simulink model "sampleModel7293_pp_1_1"  (R2018a)
settings: Solver=VariableStepAuto  StartTime=0.0  StopTime=10.0  RelTol=1e-3
undefined symbols (not defined in the file): DiscIntNeverNeededParam
libraries: simulink x367
(part 5 of 12)

== system sampleModel7293_pp_1_1/cfblk209 ==
  cfblk1 : Inport
  Action Port : ActionPort  ActionType=else
  cfblk10 : Subsystem  TreatAsAtomicUnit=on
  cfblk11 : Delay
  cfblk12 : Subsystem  TreatAsAtomicUnit=on
  cfblk13 : Delay
  cfblk3 : DiscreteTransferFcn
  cfblk4 : Subsystem  TreatAsAtomicUnit=on
  cfblk5 : simulink/Continuous/PID Controller (2DOF)  Controller=PID  TimeDomain=Discrete-time  SampleTime=-1  IntegratorMethod=Forward Euler  FilterMethod=Forward Euler  Form=Parallel  UseFilter=on  ControllerParametersSource=internal  P=1  I=1  D=0  N=100  b=1  c=1  InitialConditionSource=internal  InitialConditionForIntegrator=0  InitialConditionForFilter=0  ExternalReset=none  LimitOutput=off  UpperSaturationLimit=inf  LowerSaturationLimit=-inf  LinearizeAsGain=off  AntiWindupMode=none  Kb=1  TrackingMode=off  Kt=1  PParamMin=[]  PParamMax=[]  IParamMin=[]  IParamMax=[]  DParamMin=[]  DParamMax=[]  NParamMin=[]  NParamMax=[]  bParamMin=[]  bParamMax=[]  cParamMin=[]  cParamMax=[]  KbParamMin=[]  KbParamMax=[]  KtParamMin=[]  KtParamMax=[]  POutMin=[]  POutMax=[]  IOutMin=[]  IOutMax=[]  DOutMin=[]  DOutMax=[]  NOutMin=[]  NOutMax=[]  bOutMin=[]  bOutMax=[]  cOutMin=[]  cOutMax=[]  KbOutMin=[]  KbOutMax=[]  KtOutMin=[]  KtOutMax=[]  IntegratorOutMin=[]  IntegratorOutMax=[]  FilterOutMin=[]  FilterOutMax=[]  SumOutMin=[]  SumOutMax=[]  Sum1OutMin=[]  Sum1OutMax=[]  Sum2OutMin=[]  Sum2OutMax=[]  Sum3OutMin=[]  Sum3OutMax=[]  SumI1OutMin=[]  SumI1OutMax=[]  SumI2OutMin=[]  SumI2OutMax=[]  SumI3OutMin=[]  SumI3OutMax=[]  SumDOutMin=[]  SumDOutMax=[]  SaturationOutMin=[]  SaturationOutMax=[]  IntegratorContinuousStateAttributes=''  IntegratorStateMustResolveToSignalObject=off  IntegratorRTWStateStorageClass=Auto  FilterContinuousStateAttributes=''  FilterStateMustResolveToSignalObject=off  FilterRTWStateStorageClass=Auto  DifferentiatorICPrevScaledInput=0  DifferentiatorOutMin=[]  DifferentiatorOutMax=[]  FilterDiffOutCoefMin=[]  FilterDiffOutCoefMax=[]  SumDenOutMin=[]  SumDenOutMax=[]  SumNumOutMin=[]  SumNumOutMax=[]  ReciprocalOutMin=[]  ReciprocalOutMax=[]  DivideOutMin=[]  DivideOutMax=[]  TunerSelectOption=Transfer Function Based (PID Tuner App)
  cfblk6 : Subsystem  TreatAsAtomicUnit=on
  cfblk7 : simulink/Discrete/Difference  ICPrevInput=0.0  OutMin=[]  OutMax=[]  OutDataTypeStr=double  OutputDataTypeScalingMode=double  OutDataType=fixdt(1, 16)  OutScaling=2^-10  DoSatur=off
  cfblk8 : If  SampleTime=1
  cfblk9 : Subsystem  TreatAsAtomicUnit=on
  cyemi_{1328..1329,1341..1352} (14 alike) : DataTypeConversion  OutDataTypeStr=double
  emi_1702 : Subsystem  TreatAsAtomicUnit=on
  emi_1704 : If  IfExpression=0 <= u1
  emi_1705 : DataTypeConversion  OutDataTypeStr=double
  emi_1908 : Subsystem  TreatAsAtomicUnit=on
  emi_1910 : If  IfExpression=0 <= u1
  emi_1911 : DataTypeConversion  OutDataTypeStr=double
  emi_783 : Subsystem  TreatAsAtomicUnit=on
  emi_785 : If  IfExpression=0 <= u1
  emi_786 : DataTypeConversion  OutDataTypeStr=double
  cfblk2 : Outport
  wires:
  cfblk10/1(cfblk2) -> cfblk2/1
  cfblk7/1 -> cyemi_1342/1, cyemi_1343/1
  cfblk8/1 -> cfblk9/Action
  cfblk8/2 -> cfblk10/Action
  cyemi_1328/1 -> cfblk10/1(cfblk1)
  cyemi_1329/1 -> cfblk10/2(cfblk12)
  cfblk13/1 -> cyemi_1329/1, emi_786/1
  cyemi_1341/1 -> cfblk11/1
  cfblk5/1 -> cyemi_1341/1
  cyemi_1343/1 -> cfblk13/1
  cyemi_1344/1 -> cfblk3/1
  cfblk9/1(cfblk2) -> cyemi_1344/1
  cyemi_1346/1 -> cfblk5/1
  cfblk3/1 -> cyemi_1346/1
  cyemi_1347/1 -> cfblk5/2
  cfblk9/2(cfblk16) -> cyemi_1347/1
  cfblk1/1 -> cyemi_1348/1
  cyemi_1349/1 -> cfblk7/1
  cfblk10/3(cfblk14) -> cyemi_1349/1
  cyemi_1350/1 -> cfblk8/1
  cyemi_1351/1 -> cfblk9/1(cfblk1)
  cfblk11/1 -> cyemi_1351/1, emi_1705/1
  cyemi_1352/1 -> cfblk9/2(cfblk15)
  cfblk10/2(cfblk13) -> cyemi_1352/1
  cyemi_1345/1 -> cfblk4/1(emi_781)
  cfblk4/1(emi_782) -> cyemi_1350/1, emi_1911/1
  emi_785/1 -> cfblk4/Action
  emi_785/2 -> emi_783/Action
  emi_786/1 -> emi_785/1
  cyemi_1348/1 -> cfblk6/1(emi_1700)
  cfblk6/1(emi_1701) -> cyemi_1345/1
  emi_1704/1 -> cfblk6/Action
  emi_1704/2 -> emi_1702/Action
  emi_1705/1 -> emi_1704/1
  cyemi_1342/1 -> cfblk12/1(emi_1906)
  cfblk12/1(emi_1907) -> cyemi_1328/1
  emi_1910/1 -> cfblk12/Action
  emi_1910/2 -> emi_1908/Action
  emi_1911/1 -> emi_1910/1

== system sampleModel7293_pp_1_1/cfblk210 ==
  cfblk1 : Inport
  cfblk14 : Inport  Port=2
  cfblk15 : Inport  Port=3
  Action Port : ActionPort  ActionType=then
  cfblk10 : simulink/Continuous/PID Controller (2DOF)  Controller=PID  TimeDomain=Discrete-time  SampleTime=-1  IntegratorMethod=Forward Euler  FilterMethod=Forward Euler  Form=Parallel  UseFilter=on  ControllerParametersSource=internal  P=1  I=1  D=0  N=100  b=1  c=1  InitialConditionSource=internal  InitialConditionForIntegrator=0  InitialConditionForFilter=0  ExternalReset=none  LimitOutput=off  UpperSaturationLimit=inf  LowerSaturationLimit=-inf  LinearizeAsGain=off  AntiWindupMode=none  Kb=1  TrackingMode=off  Kt=1  PParamMin=[]  PParamMax=[]  IParamMin=[]  IParamMax=[]  DParamMin=[]  DParamMax=[]  NParamMin=[]  NParamMax=[]  bParamMin=[]  bParamMax=[]  cParamMin=[]  cParamMax=[]  KbParamMin=[]  KbParamMax=[]  KtParamMin=[]  KtParamMax=[]  POutMin=[]  POutMax=[]  IOutMin=[]  IOutMax=[]  DOutMin=[]  DOutMax=[]  NOutMin=[]  NOutMax=[]  bOutMin=[]  bOutMax=[]  cOutMin=[]  cOutMax=[]  KbOutMin=[]  KbOutMax=[]  KtOutMin=[]  KtOutMax=[]  IntegratorOutMin=[]  IntegratorOutMax=[]  FilterOutMin=[]  FilterOutMax=[]  SumOutMin=[]  SumOutMax=[]  Sum1OutMin=[]  Sum1OutMax=[]  Sum2OutMin=[]  Sum2OutMax=[]  Sum3OutMin=[]  Sum3OutMax=[]  SumI1OutMin=[]  SumI1OutMax=[]  SumI2OutMin=[]  SumI2OutMax=[]  SumI3OutMin=[]  SumI3OutMax=[]  SumDOutMin=[]  SumDOutMax=[]  SaturationOutMin=[]  SaturationOutMax=[]  IntegratorContinuousStateAttributes=''  IntegratorStateMustResolveToSignalObject=off  IntegratorRTWStateStorageClass=Auto  FilterContinuousStateAttributes=''  FilterStateMustResolveToSignalObject=off  FilterRTWStateStorageClass=Auto  DifferentiatorICPrevScaledInput=0  DifferentiatorOutMin=[]  DifferentiatorOutMax=[]  FilterDiffOutCoefMin=[]  FilterDiffOutCoefMax=[]  SumDenOutMin=[]  SumDenOutMax=[]  SumNumOutMin=[]  SumNumOutMax=[]  ReciprocalOutMin=[]  ReciprocalOutMax=[]  DivideOutMin=[]  DivideOutMax=[]  TunerSelectOption=Transfer Function Based (PID Tuner App)
  cfblk11 : simulink/Discrete/Transfer Fcn First Order  PoleZ=0.95  ICPrevOutput=0.0  DoSatur=off
      settings: SourceProductName=Simulink
  cfblk12 : simulink/Discrete/Tapped Delay  vinit=0.0  samptime=-1  NumDelays=1  DelayOrder=Oldest  includeCurrent=off
  cfblk13 : If  SampleTime=1
  cfblk17 : Subsystem  TreatAsAtomicUnit=on
  cfblk18 : Subsystem  TreatAsAtomicUnit=on
  cfblk19 : Delay
  cfblk20 : Delay
  cfblk21 : Delay
  cfblk3 : DiscreteZeroPole  Poles=[0 0.5]  Gain=1  SampleTime=-1
  cfblk4 : DiscreteFir
  cfblk5 : simulink/Discrete/Transfer Fcn Lead or Lag  PoleZ=0.95  ZeroZ=0.75  ICPrevOutput=0.0  ICPrevInput=0.0  DoSatur=off
      settings: SourceProductName=Simulink  SourceProductBaseCode=SL
  cfblk6 : simulink/Discrete/Difference  ICPrevInput=0.0  OutMin=[]  OutMax=[]  OutDataTypeStr=double  OutputDataTypeScalingMode=double  OutDataType=fixdt(1, 16)  OutScaling=2^-10  DoSatur=off
  cfblk7 : DiscreteStateSpace  SampleTime=-1
  cfblk8 : Delay  ShowEnablePort=on
      settings: InputPortMap=u0,e6
  cfblk9 : DiscreteTransferFcn
  cyemi_{1371..1377,1383..1385,1395..1405} (21 alike) : DataTypeConversion  OutDataTypeStr=double
  cfblk2 : Outport
  cfblk16 : Outport  Port=2
  wires:
  cfblk14/1 -> cyemi_1377/1, cyemi_1404/1
  cfblk17/1(cfblk2) -> cyemi_1374/1, cyemi_1384/1
  cfblk10/1 -> cfblk2/1, cyemi_1400/1
  cfblk12/1 -> cyemi_1373/1, cyemi_1397/1
  cfblk9/1 -> cyemi_1399/1, cyemi_1401/1
  cfblk3/1 -> cfblk16/1
  cfblk13/1 -> cfblk17/Action
  cfblk13/2 -> cfblk18/Action
  cyemi_1371/1 -> cfblk10/1
  cfblk8/1 -> cyemi_1371/1
  cyemi_1372/1 -> cfblk10/2
  cfblk20/1 -> cyemi_1372/1
  cyemi_1373/1 -> cfblk11/1
  cyemi_1374/1 -> cfblk12/1
  cyemi_1375/1 -> cfblk13/1
  cfblk5/1 -> cyemi_1375/1
  cyemi_1376/1 -> cfblk17/1(cfblk1)
  cfblk6/1 -> cyemi_1376/1
  cyemi_1377/1 -> cfblk17/2(cfblk8)
  cyemi_1383/1 -> cfblk18/1(cfblk1)
  cfblk19/1 -> cyemi_1383/1
  cyemi_1384/1 -> cfblk18/2(cfblk12)
  cyemi_1385/1 -> cfblk18/3(cfblk13)
  cfblk21/1 -> cyemi_1385/1
  cyemi_1395/1 -> cfblk19/1
  cfblk11/1 -> cyemi_1395/1
  cyemi_1396/1 -> cfblk20/1
  cfblk18/1(cfblk2) -> cyemi_1396/1
  cyemi_1397/1 -> cfblk21/1
  cyemi_1398/1 -> cfblk3/1
  cfblk1/1 -> cyemi_1398/1
  cyemi_1399/1 -> cfblk4/1
  cyemi_1400/1 -> cfblk5/1
  cyemi_1401/1 -> cfblk6/1
  cyemi_1402/1 -> cfblk7/1
  cfblk4/1 -> cyemi_1402/1
  cyemi_1403/1 -> cfblk8/1
  cfblk7/1 -> cyemi_1403/1
  cyemi_1404/1 -> cfblk8/2
  cyemi_1405/1 -> cfblk9/1
  cfblk15/1 -> cyemi_1405/1

== system sampleModel7293_pp_1_1/cfblk211 ==
  cfblk1 : Inport
  Action Port : ActionPort  ActionType=else
  cfblk3 : DiscreteTransferFcn
  cfblk4 : Delay
  cfblk5 : Subsystem  TreatAsAtomicUnit=on
  cfblk8 : Delay
  cyemi_{1407..1410} (4 alike) : DataTypeConversion  OutDataTypeStr=double
  emi_1859 : Subsystem  TreatAsAtomicUnit=on
  emi_1861 : If  IfExpression=Inf <= u1
  emi_1862 : DataTypeConversion  OutDataTypeStr=double
  cfblk2 : Outport
  cfblk6 : Outport  Port=2
  cfblk7 : Outport  Port=3
  wires:
  cfblk3/1 -> cfblk2/1
  cfblk1/1 -> cfblk6/1
  cfblk4/1 -> cyemi_1407/1, cyemi_1409/1
  cyemi_1407/1 -> cfblk3/1
  cyemi_1408/1 -> cfblk4/1
  cfblk8/1 -> cyemi_1408/1, emi_1862/1
  cyemi_1410/1 -> cfblk8/1
  cyemi_1409/1 -> cfblk5/1(emi_1857)
  cfblk5/1(emi_1858) -> cyemi_1410/1, cfblk7/1
  emi_1861/1 -> cfblk5/Action
  emi_1861/2 -> emi_1859/Action
  emi_1862/1 -> emi_1861/1

== system sampleModel7293_pp_1_1/cfblk212 ==
  cfblk1 : Inport
  cfblk8 : Inport  Port=2
  cfblk9 : Inport  Port=3
  Action Port : ActionPort  ActionType=then
  cfblk10 : Delay
  cfblk3 : Delay  ShowEnablePort=on
      settings: InputPortMap=u0,e6
  cfblk4 : simulink/Discrete/Transfer Fcn Lead or Lag  PoleZ=0.95  ZeroZ=0.75  ICPrevOutput=0.0  ICPrevInput=0.0  DoSatur=off
      settings: SourceProductName=Simulink  SourceProductBaseCode=SL
  cfblk5 : Delay
  cfblk6 : Delay  ShowEnablePort=on
      settings: InputPortMap=u0,e6
  cfblk7 : simulink/Continuous/PID Controller  Controller=PID  TimeDomain=Discrete-time  SampleTime=-1  IntegratorMethod=Forward Euler  FilterMethod=Forward Euler  Form=Parallel  UseFilter=on  ControllerParametersSource=internal  P=1  I=1  D=0  N=100  InitialConditionSource=internal  InitialConditionForIntegrator=0  InitialConditionForFilter=0  ExternalReset=none  LimitOutput=off  UpperSaturationLimit=inf  LowerSaturationLimit=-inf  LinearizeAsGain=off  AntiWindupMode=none  Kb=1  TrackingMode=off  Kt=1  PParamMin=[]  PParamMax=[]  IParamMin=[]  IParamMax=[]  DParamMin=[]  DParamMax=[]  NParamMin=[]  NParamMax=[]  KbParamMin=[]  KbParamMax=[]  KtParamMin=[]  KtParamMax=[]  POutMin=[]  POutMax=[]  IOutMin=[]  IOutMax=[]  DOutMin=[]  DOutMax=[]  NOutMin=[]  NOutMax=[]  KbOutMin=[]  KbOutMax=[]  KtOutMin=[]  KtOutMax=[]  IntegratorOutMin=[]  IntegratorOutMax=[]  FilterOutMin=[]  FilterOutMax=[]  SumOutMin=[]  SumOutMax=[]  SumI1OutMin=[]  SumI1OutMax=[]  SumI2OutMin=[]  SumI2OutMax=[]  SumI3OutMin=[]  SumI3OutMax=[]  SumDOutMin=[]  SumDOutMax=[]  SaturationOutMin=[]  SaturationOutMax=[]  IntegratorContinuousStateAttributes=''  IntegratorStateMustResolveToSignalObject=off  IntegratorRTWStateStorageClass=Auto  FilterContinuousStateAttributes=''  FilterStateMustResolveToSignalObject=off  FilterRTWStateStorageClass=Auto  DifferentiatorICPrevScaledInput=0  DifferentiatorOutMin=[]  DifferentiatorOutMax=[]  FilterDiffOutCoefMin=[]  FilterDiffOutCoefMax=[]  SumDenOutMin=[]  SumDenOutMax=[]  SumNumOutMin=[]  SumNumOutMax=[]  ReciprocalOutMin=[]  ReciprocalOutMax=[]  DivideOutMin=[]  DivideOutMax=[]  TunerSelectOption=Transfer Function Based (PID Tuner App)
  cyemi_{1414..1421} (8 alike) : DataTypeConversion  OutDataTypeStr=double
  cfblk2 : Outport
  wires:
  cfblk9/1 -> cfblk2/1
  cyemi_1414/1 -> cfblk10/1
  cfblk7/1 -> cyemi_1414/1
  cyemi_1415/1 -> cfblk3/1
  cfblk4/1 -> cyemi_1415/1
  cyemi_1416/1 -> cfblk3/2
  cfblk10/1 -> cyemi_1416/1
  cyemi_1417/1 -> cfblk4/1
  cfblk1/1 -> cyemi_1417/1
  cyemi_1418/1 -> cfblk5/1
  cfblk6/1 -> cyemi_1418/1
  cyemi_1419/1 -> cfblk6/1
  cfblk8/1 -> cyemi_1419/1
  cyemi_1420/1 -> cfblk6/2
  cfblk3/1 -> cyemi_1420/1
  cyemi_1421/1 -> cfblk7/1
  cfblk5/1 -> cyemi_1421/1

== system sampleModel7293_pp_1_1/cfblk213 ==
  cfblk1 : Inport
  cfblk12 : Inport  Port=2
  Action Port : ActionPort  ActionType=else
  cfblk10 : Subsystem  TreatAsAtomicUnit=on
  cfblk11 : If  SampleTime=1
  cfblk14 : Subsystem  TreatAsAtomicUnit=on
  cfblk15 : Subsystem  TreatAsAtomicUnit=on
  cfblk16 : Subsystem  TreatAsAtomicUnit=on
  cfblk17 : Delay
  cfblk3 : DiscreteIntegrator  SampleTime=-1  OutDataTypeStr=double  ICPrevOutput=DiscIntNeverNeededParam  ICPrevScaledInput=DiscIntNeverNeededParam
  cfblk4 : simulink/Discrete/Tapped Delay  vinit=0.0  samptime=-1  NumDelays=1  DelayOrder=Oldest  includeCurrent=off
  cfblk5 : simulink/Discrete/Transfer Fcn Real Zero  ZeroZ=0.75  ICPrevInput=0.0  DoSatur=off
      settings: SourceProductName=Simulink  SourceProductBaseCode=SL
  cfblk6 : simulink/Continuous/PID Controller  Controller=PID  TimeDomain=Discrete-time  SampleTime=-1  IntegratorMethod=Forward Euler  FilterMethod=Forward Euler  Form=Parallel  UseFilter=on  ControllerParametersSource=internal  P=1  I=1  D=0  N=100  InitialConditionSource=internal  InitialConditionForIntegrator=0  InitialConditionForFilter=0  ExternalReset=none  LimitOutput=off  UpperSaturationLimit=inf  LowerSaturationLimit=-inf  LinearizeAsGain=off  AntiWindupMode=none  Kb=1  TrackingMode=off  Kt=1  PParamMin=[]  PParamMax=[]  IParamMin=[]  IParamMax=[]  DParamMin=[]  DParamMax=[]  NParamMin=[]  NParamMax=[]  KbParamMin=[]  KbParamMax=[]  KtParamMin=[]  KtParamMax=[]  POutMin=[]  POutMax=[]  IOutMin=[]  IOutMax=[]  DOutMin=[]  DOutMax=[]  NOutMin=[]  NOutMax=[]  KbOutMin=[]  KbOutMax=[]  KtOutMin=[]  KtOutMax=[]  IntegratorOutMin=[]  IntegratorOutMax=[]  FilterOutMin=[]  FilterOutMax=[]  SumOutMin=[]  SumOutMax=[]  SumI1OutMin=[]  SumI1OutMax=[]  SumI2OutMin=[]  SumI2OutMax=[]  SumI3OutMin=[]  SumI3OutMax=[]  SumDOutMin=[]  SumDOutMax=[]  SaturationOutMin=[]  SaturationOutMax=[]  IntegratorContinuousStateAttributes=''  IntegratorStateMustResolveToSignalObject=off  IntegratorRTWStateStorageClass=Auto  FilterContinuousStateAttributes=''  FilterStateMustResolveToSignalObject=off  FilterRTWStateStorageClass=Auto  DifferentiatorICPrevScaledInput=0  DifferentiatorOutMin=[]  DifferentiatorOutMax=[]  FilterDiffOutCoefMin=[]  FilterDiffOutCoefMax=[]  SumDenOutMin=[]  SumDenOutMax=[]  SumNumOutMin=[]  SumNumOutMax=[]  ReciprocalOutMin=[]  ReciprocalOutMax=[]  DivideOutMin=[]  DivideOutMax=[]  TunerSelectOption=Transfer Function Based (PID Tuner App)
  cfblk7 : Delay  DelayLengthSource=Input port
      settings: InputPortMap=u0,p1
  cfblk8 : simulink/Continuous/PID Controller  Controller=PID  TimeDomain=Discrete-time  SampleTime=-1  IntegratorMethod=Forward Euler  FilterMethod=Forward Euler  Form=Parallel  UseFilter=on  ControllerParametersSource=internal  P=1  I=1  D=0  N=100  InitialConditionSource=internal  InitialConditionForIntegrator=0  InitialConditionForFilter=0  ExternalReset=none  LimitOutput=off  UpperSaturationLimit=inf  LowerSaturationLimit=-inf  LinearizeAsGain=off  AntiWindupMode=none  Kb=1  TrackingMode=off  Kt=1  PParamMin=[]  PParamMax=[]  IParamMin=[]  IParamMax=[]  DParamMin=[]  DParamMax=[]  NParamMin=[]  NParamMax=[]  KbParamMin=[]  KbParamMax=[]  KtParamMin=[]  KtParamMax=[]  POutMin=[]  POutMax=[]  IOutMin=[]  IOutMax=[]  DOutMin=[]  DOutMax=[]  NOutMin=[]  NOutMax=[]  KbOutMin=[]  KbOutMax=[]  KtOutMin=[]  KtOutMax=[]  IntegratorOutMin=[]  IntegratorOutMax=[]  FilterOutMin=[]  FilterOutMax=[]  SumOutMin=[]  SumOutMax=[]  SumI1OutMin=[]  SumI1OutMax=[]  SumI2OutMin=[]  SumI2OutMax=[]  SumI3OutMin=[]  SumI3OutMax=[]  SumDOutMin=[]  SumDOutMax=[]  SaturationOutMin=[]  SaturationOutMax=[]  IntegratorContinuousStateAttributes=''  IntegratorStateMustResolveToSignalObject=off  IntegratorRTWStateStorageClass=Auto  FilterContinuousStateAttributes=''  FilterStateMustResolveToSignalObject=off  FilterRTWStateStorageClass=Auto  DifferentiatorICPrevScaledInput=0  DifferentiatorOutMin=[]  DifferentiatorOutMax=[]  FilterDiffOutCoefMin=[]  FilterDiffOutCoefMax=[]  SumDenOutMin=[]  SumDenOutMax=[]  SumNumOutMin=[]  SumNumOutMax=[]  ReciprocalOutMin=[]  ReciprocalOutMax=[]  DivideOutMin=[]  DivideOutMax=[]  TunerSelectOption=Transfer Function Based (PID Tuner App)
  cfblk9 : simulink/Continuous/PID Controller (2DOF)  Controller=PID  TimeDomain=Discrete-time  SampleTime=-1  IntegratorMethod=Forward Euler  FilterMethod=Forward Euler  Form=Parallel  UseFilter=on  ControllerParametersSource=internal  P=1  I=1  D=0  N=100  b=1  c=1  InitialConditionSource=internal  InitialConditionForIntegrator=0  InitialConditionForFilter=0  ExternalReset=none  LimitOutput=off  UpperSaturationLimit=inf  LowerSaturationLimit=-inf  LinearizeAsGain=off  AntiWindupMode=none  Kb=1  TrackingMode=off  Kt=1  PParamMin=[]  PParamMax=[]  IParamMin=[]  IParamMax=[]  DParamMin=[]  DParamMax=[]  NParamMin=[]  NParamMax=[]  bParamMin=[]  bParamMax=[]  cParamMin=[]  cParamMax=[]  KbParamMin=[]  KbParamMax=[]  KtParamMin=[]  KtParamMax=[]  POutMin=[]  POutMax=[]  IOutMin=[]  IOutMax=[]  DOutMin=[]  DOutMax=[]  NOutMin=[]  NOutMax=[]  bOutMin=[]  bOutMax=[]  cOutMin=[]  cOutMax=[]  KbOutMin=[]  KbOutMax=[]  KtOutMin=[]  KtOutMax=[]  IntegratorOutMin=[]  IntegratorOutMax=[]  FilterOutMin=[]  FilterOutMax=[]  SumOutMin=[]  SumOutMax=[]  Sum1OutMin=[]  Sum1OutMax=[]  Sum2OutMin=[]  Sum2OutMax=[]  Sum3OutMin=[]  Sum3OutMax=[]  SumI1OutMin=[]  SumI1OutMax=[]  SumI2OutMin=[]  SumI2OutMax=[]  SumI3OutMin=[]  SumI3OutMax=[]  SumDOutMin=[]  SumDOutMax=[]  SaturationOutMin=[]  SaturationOutMax=[]  IntegratorContinuousStateAttributes=''  IntegratorStateMustResolveToSignalObject=off  IntegratorRTWStateStorageClass=Auto  FilterContinuousStateAttributes=''  FilterStateMustResolveToSignalObject=off  FilterRTWStateStorageClass=Auto  DifferentiatorICPrevScaledInput=0  DifferentiatorOutMin=[]  DifferentiatorOutMax=[]  FilterDiffOutCoefMin=[]  FilterDiffOutCoefMax=[]  SumDenOutMin=[]  SumDenOutMax=[]  SumNumOutMin=[]  SumNumOutMax=[]  ReciprocalOutMin=[]  ReciprocalOutMax=[]  DivideOutMin=[]  DivideOutMax=[]  TunerSelectOption=Transfer Function Based (PID Tuner App)
  cyemi_{1424..1428,1447..1448,1457..1467} (18 alike) : DataTypeConversion  OutDataTypeStr=double
  emi_1332 : Subsystem  TreatAsAtomicUnit=on
  emi_1334 : If  IfExpression=0 <= u1
  emi_1335 : DataTypeConversion  OutDataTypeStr=double
  emi_1360 : Subsystem  TreatAsAtomicUnit=on
  emi_1362 : If  IfExpression=0 <= u1
  emi_1363 : DataTypeConversion  OutDataTypeStr=double
  cfblk2 : Outport
  cfblk13 : Outport  Port=2
  wires:
  cfblk4/1 -> cyemi_1424/1, cyemi_1428/1, cyemi_1448/1
  cfblk9/1 -> cfblk13/1
  cfblk6/1 -> cfblk2/1
  cfblk1/1 -> cyemi_1447/1, cyemi_1467/1
  cfblk12/1 -> cyemi_1425/1, cyemi_1426/1
  cfblk11/1 -> cfblk14/Action
  cfblk11/2 -> cfblk15/Action
  cyemi_1425/1 -> cfblk11/1
  cyemi_1426/1 -> cfblk14/1(cfblk1)
  cyemi_1427/1 -> cfblk14/2(cfblk13)
  cfblk17/1 -> cyemi_1427/1
  cyemi_1428/1 -> cfblk14/3(cfblk14)
  cyemi_1447/1 -> cfblk15/1(cfblk1)
  cyemi_1448/1 -> cfblk15/2(cfblk9)
  cyemi_1458/1 -> cfblk17/1
  cfblk5/1 -> cyemi_1458/1
  cyemi_1459/1 -> cfblk3/1
  cfblk15/1(cfblk2) -> cyemi_1459/1
  cyemi_1460/1 -> cfblk4/1
  cyemi_1461/1 -> cfblk5/1
  cfblk14/1(cfblk2) -> cyemi_1461/1
  cyemi_1462/1 -> cfblk6/1
  cfblk14/2(cfblk15) -> cyemi_1462/1
  cyemi_1463/1 -> cfblk7/1
  cfblk15/2(cfblk10) -> cyemi_1463/1
  cyemi_1464/1 -> cfblk7/2
  cfblk3/1 -> cyemi_1464/1, emi_1335/1
  cyemi_1465/1 -> cfblk8/1
  cfblk7/1 -> cyemi_1465/1
  cyemi_1466/1 -> cfblk9/1
  cfblk8/1 -> cyemi_1466/1
  cyemi_1467/1 -> cfblk9/2
  cyemi_1424/1 -> cfblk10/1(emi_1330)
  cfblk10/1(emi_1331) -> cyemi_1457/1, emi_1363/1
  emi_1334/1 -> cfblk10/Action
  emi_1334/2 -> emi_1332/Action
  emi_1335/1 -> emi_1334/1
  cyemi_1457/1 -> cfblk16/1(emi_1358)
  cfblk16/1(emi_1359) -> cyemi_1460/1
  emi_1362/1 -> cfblk16/Action
  emi_1362/2 -> emi_1360/Action
  emi_1363/1 -> emi_1362/1

== system sampleModel7293_pp_1_1/cfblk214 ==
  emi_1443 : Inport
  Action Port : ActionPort  ActionType=then
  cfblk214 : Delay  SampleTime=1
  emi_1444 : Outport
  wires:
  emi_1443/1 -> cfblk214/1
  cfblk214/1 -> emi_1444/1

== system sampleModel7293_pp_1_1/cfblk215 ==
  emi_1515 : Inport
  Action Port : ActionPort  ActionType=then
  cfblk215 : Delay  SampleTime=1
  emi_1516 : Outport
  wires:
  emi_1515/1 -> cfblk215/1
  cfblk215/1 -> emi_1516/1

== system sampleModel7293_pp_1_1/cfblk218 ==
  emi_1786 : Inport
  Action Port : ActionPort  ActionType=then
  cfblk218 : Delay  SampleTime=1
  emi_1787 : Outport
  wires:
  emi_1786/1 -> cfblk218/1
  cfblk218/1 -> emi_1787/1

== system sampleModel7293_pp_1_1/cfblk219 ==
  emi_1337 : Inport
  Action Port : ActionPort  ActionType=then
  cfblk219 : Delay  SampleTime=1
  emi_1338 : Outport
  wires:
  emi_1337/1 -> cfblk219/1
  cfblk219/1 -> emi_1338/1

== system sampleModel7293_pp_1_1/cfblk22 ==
  emi_702 : Inport
  emi_703 : Inport  Port=2
  Action Port : ActionPort  ActionType=then
  cfblk22 : simulink/Continuous/PID Controller (2DOF)  Controller=PID  TimeDomain=Discrete-time  SampleTime=1  IntegratorMethod=Forward Euler  FilterMethod=Forward Euler  Form=Parallel  UseFilter=on  ControllerParametersSource=internal  P=1  I=1  D=0  N=100  b=1  c=1  InitialConditionSource=internal  InitialConditionForIntegrator=0  InitialConditionForFilter=0  ExternalReset=none  LimitOutput=off  UpperSaturationLimit=inf  LowerSaturationLimit=-inf  LinearizeAsGain=off  AntiWindupMode=none  Kb=1  TrackingMode=off  Kt=1  PParamMin=[]  PParamMax=[]  IParamMin=[]  IParamMax=[]  DParamMin=[]  DParamMax=[]  NParamMin=[]  NParamMax=[]  bParamMin=[]  bParamMax=[]  cParamMin=[]  cParamMax=[]  KbParamMin=[]  KbParamMax=[]  KtParamMin=[]  KtParamMax=[]  POutMin=[]  POutMax=[]  IOutMin=[]  IOutMax=[]  DOutMin=[]  DOutMax=[]  NOutMin=[]  NOutMax=[]  bOutMin=[]  bOutMax=[]  cOutMin=[]  cOutMax=[]  KbOutMin=[]  KbOutMax=[]  KtOutMin=[]  KtOutMax=[]  IntegratorOutMin=[]  IntegratorOutMax=[]  FilterOutMin=[]  FilterOutMax=[]  SumOutMin=[]  SumOutMax=[]  Sum1OutMin=[]  Sum1OutMax=[]  Sum2OutMin=[]  Sum2OutMax=[]  Sum3OutMin=[]  Sum3OutMax=[]  SumI1OutMin=[]  SumI1OutMax=[]  SumI2OutMin=[]  SumI2OutMax=[]  SumI3OutMin=[]  SumI3OutMax=[]  SumDOutMin=[]  SumDOutMax=[]  SaturationOutMin=[]  SaturationOutMax=[]  IntegratorContinuousStateAttributes=''  IntegratorStateMustResolveToSignalObject=off  IntegratorRTWStateStorageClass=Auto  FilterContinuousStateAttributes=''  FilterStateMustResolveToSignalObject=off  FilterRTWStateStorageClass=Auto  DifferentiatorICPrevScaledInput=0  DifferentiatorOutMin=[]  DifferentiatorOutMax=[]  FilterDiffOutCoefMin=[]  FilterDiffOutCoefMax=[]  SumDenOutMin=[]  SumDenOutMax=[]  SumNumOutMin=[]  SumNumOutMax=[]  ReciprocalOutMin=[]  ReciprocalOutMax=[]  DivideOutMin=[]  DivideOutMax=[]  TunerSelectOption=Transfer Function Based (PID Tuner App)
  emi_704 : Outport
  wires:
  emi_702/1 -> cfblk22/1
  emi_703/1 -> cfblk22/2
  cfblk22/1 -> emi_704/1

== system sampleModel7293_pp_1_1/cfblk220 ==
  emi_945 : Inport
  Action Port : ActionPort  ActionType=then
  cfblk220 : Delay  SampleTime=1
  emi_946 : Outport
  wires:
  emi_945/1 -> cfblk220/1
  cfblk220/1 -> emi_946/1

== system sampleModel7293_pp_1_1/cfblk227 ==
  emi_1393 : Inport
  Action Port : ActionPort  ActionType=then
  cfblk227 : Delay  SampleTime=1
  emi_1394 : Outport
  wires:
  emi_1393/1 -> cfblk227/1
  cfblk227/1 -> emi_1394/1

== system sampleModel7293_pp_1_1/cfblk230 ==
  emi_739 : Inport
  Action Port : ActionPort  ActionType=then
  cfblk230 : Delay  SampleTime=1
  emi_740 : Outport
  wires:
  emi_739/1 -> cfblk230/1
  cfblk230/1 -> emi_740/1

== system sampleModel7293_pp_1_1/cfblk231 ==
  emi_436 : Inport
  Action Port : ActionPort  ActionType=then
  cfblk231 : Delay  SampleTime=1
  emi_437 : Outport
  wires:
  emi_436/1 -> cfblk231/1
  cfblk231/1 -> emi_437/1

== system sampleModel7293_pp_1_1/cfblk233 ==
  emi_1543 : Inport
  Action Port : ActionPort  ActionType=then
  cfblk233 : Delay  SampleTime=1
  emi_1544 : Outport
  wires:
  emi_1543/1 -> cfblk233/1
  cfblk233/1 -> emi_1544/1

== system sampleModel7293_pp_1_1/cfblk239 ==
  emi_373 : Inport
  Action Port : ActionPort  ActionType=then
  cfblk239 : Delay  SampleTime=1
  emi_374 : Outport
  wires:
  emi_373/1 -> cfblk239/1
  cfblk239/1 -> emi_374/1

== system sampleModel7293_pp_1_1/cfblk240 ==
  emi_329 : Inport
  Action Port : ActionPort  ActionType=then
  cfblk240 : Delay  SampleTime=1
  emi_330 : Outport
  wires:
  emi_329/1 -> cfblk240/1
  cfblk240/1 -> emi_330/1

== system sampleModel7293_pp_1_1/cfblk247 ==
  emi_401 : Inport
  Action Port : ActionPort  ActionType=then
  cfblk247 : Delay  SampleTime=1
  emi_402 : Outport
  wires:
  emi_401/1 -> cfblk247/1
  cfblk247/1 -> emi_402/1

== system sampleModel7293_pp_1_1/cfblk255 ==
  emi_1913 : Inport
  Action Port : ActionPort  ActionType=then
  cfblk255 : Delay  SampleTime=1
  emi_1914 : Outport
  wires:
  emi_1913/1 -> cfblk255/1
  cfblk255/1 -> emi_1914/1

== system sampleModel7293_pp_1_1/cfblk256 ==
  emi_143 : Inport
  Action Port : ActionPort  ActionType=then
  cfblk256 : Delay  SampleTime=1
  emi_144 : Outport
  wires:
  emi_143/1 -> cfblk256/1
  cfblk256/1 -> emi_144/1

== system sampleModel7293_pp_1_1/cfblk259 ==
  emi_882 : Inport
  Action Port : ActionPort  ActionType=then
  cfblk259 : Delay  SampleTime=1
  emi_883 : Outport
  wires:
  emi_882/1 -> cfblk259/1
  cfblk259/1 -> emi_883/1

== system sampleModel7293_pp_1_1/cfblk268 ==
  emi_1878 : Inport
  Action Port : ActionPort  ActionType=then
  cfblk268 : Delay  SampleTime=1
  emi_1879 : Outport
  wires:
  emi_1878/1 -> cfblk268/1
  cfblk268/1 -> emi_1879/1

== system sampleModel7293_pp_1_1/cfblk273 ==
  emi_465 : Inport
  Action Port : ActionPort  ActionType=then
  cfblk273 : DataTypeConversion  OutDataTypeStr=double
  emi_466 : Outport
  wires:
  emi_465/1 -> cfblk273/1
  cfblk273/1 -> emi_466/1

== system sampleModel7293_pp_1_1/cfblk277 ==
  emi_1742 : Inport
  Action Port : ActionPort  ActionType=then
  cfblk277 : DataTypeConversion  OutDataTypeStr=double
  emi_1743 : Outport
  wires:
  emi_1742/1 -> cfblk277/1
  cfblk277/1 -> emi_1743/1

== system sampleModel7293_pp_1_1/cfblk29 ==
  emi_457 : Inport
  emi_458 : Inport  Port=2
  Action Port : ActionPort  ActionType=then
  cfblk29 : Delay  DelayLengthSource=Input port  SampleTime=1
      settings: InputPortMap=u0,p1
  emi_459 : Outport
  wires:
  emi_457/1 -> cfblk29/1
  emi_458/1 -> cfblk29/2
  cfblk29/1 -> emi_459/1

== system sampleModel7293_pp_1_1/cfblk32 ==
  emi_480 : Inport
  Action Port : ActionPort  ActionType=then
  cfblk32 : UnitDelay
  emi_481 : Outport
  wires:
  emi_480/1 -> cfblk32/1
  cfblk32/1 -> emi_481/1

== system sampleModel7293_pp_1_1/cfblk33 ==
  emi_868 : Inport
  Action Port : ActionPort  ActionType=then
  cfblk33 : simulink/Continuous/PID Controller  Controller=PID  TimeDomain=Discrete-time  SampleTime=1  IntegratorMethod=Forward Euler  FilterMethod=Forward Euler  Form=Parallel  UseFilter=on  ControllerParametersSource=internal  P=1  I=1  D=0  N=100  InitialConditionSource=internal  InitialConditionForIntegrator=0  InitialConditionForFilter=0  ExternalReset=none  LimitOutput=off  UpperSaturationLimit=inf  LowerSaturationLimit=-inf  LinearizeAsGain=off  AntiWindupMode=none  Kb=1  TrackingMode=off  Kt=1  PParamMin=[]  PParamMax=[]  IParamMin=[]  IParamMax=[]  DParamMin=[]  DParamMax=[]  NParamMin=[]  NParamMax=[]  KbParamMin=[]  KbParamMax=[]  KtParamMin=[]  KtParamMax=[]  POutMin=[]  POutMax=[]  IOutMin=[]  IOutMax=[]  DOutMin=[]  DOutMax=[]  NOutMin=[]  NOutMax=[]  KbOutMin=[]  KbOutMax=[]  KtOutMin=[]  KtOutMax=[]  IntegratorOutMin=[]  IntegratorOutMax=[]  FilterOutMin=[]  FilterOutMax=[]  SumOutMin=[]  SumOutMax=[]  SumI1OutMin=[]  SumI1OutMax=[]  SumI2OutMin=[]  SumI2OutMax=[]  SumI3OutMin=[]  SumI3OutMax=[]  SumDOutMin=[]  SumDOutMax=[]  SaturationOutMin=[]  SaturationOutMax=[]  IntegratorContinuousStateAttributes=''  IntegratorStateMustResolveToSignalObject=off  IntegratorRTWStateStorageClass=Auto  FilterContinuousStateAttributes=''  FilterStateMustResolveToSignalObject=off  FilterRTWStateStorageClass=Auto  DifferentiatorICPrevScaledInput=0  DifferentiatorOutMin=[]  DifferentiatorOutMax=[]  FilterDiffOutCoefMin=[]  FilterDiffOutCoefMax=[]  SumDenOutMin=[]  SumDenOutMax=[]  SumNumOutMin=[]  SumNumOutMax=[]  ReciprocalOutMin=[]  ReciprocalOutMax=[]  DivideOutMin=[]  DivideOutMax=[]  TunerSelectOption=Transfer Function Based (PID Tuner App)
  emi_869 : Outport
  wires:
  emi_868/1 -> cfblk33/1
  cfblk33/1 -> emi_869/1

== system sampleModel7293_pp_1_1/cfblk39 ==
  emi_753 : Inport
  Action Port : ActionPort  ActionType=then
  cfblk39 : simulink/Discrete/Transfer Fcn Real Zero  ZeroZ=0.75  ICPrevInput=0.0  DoSatur=off
      settings: SourceProductName=Simulink  SourceProductBaseCode=SL
  emi_754 : Outport
  wires:
  emi_753/1 -> cfblk39/1
  cfblk39/1 -> emi_754/1

== system sampleModel7293_pp_1_1/cfblk40 ==
  emi_1294 : Inport
  Action Port : ActionPort  ActionType=then
  cfblk40 : DiscreteFir  SampleTime=1
  emi_1295 : Outport
  wires:
  emi_1294/1 -> cfblk40/1
  cfblk40/1 -> emi_1295/1

== system sampleModel7293_pp_1_1/cfblk41 ==
  emi_1036 : Inport
  Action Port : ActionPort  ActionType=then
  cfblk41 : simulink/Discrete/Transfer Fcn Real Zero  ZeroZ=0.75  ICPrevInput=0.0  DoSatur=off
      settings: SourceProductName=Simulink  SourceProductBaseCode=SL
  emi_1037 : Outport
  wires:
  emi_1036/1 -> cfblk41/1
  cfblk41/1 -> emi_1037/1

== system sampleModel7293_pp_1_1/cfblk45 ==
  emi_931 : Inport
  Action Port : ActionPort  ActionType=then
  cfblk45 : UnitDelay
  emi_932 : Outport
  wires:
  emi_931/1 -> cfblk45/1
  cfblk45/1 -> emi_932/1

== system sampleModel7293_pp_1_1/cfblk52 ==
  emi_1478 : Inport
  emi_1479 : Inport  Port=2
  Action Port : ActionPort  ActionType=then
  cfblk52 : Delay  DelayLengthSource=Input port  SampleTime=1
      settings: InputPortMap=u0,p1
  emi_1480 : Outport
  wires:
  emi_1478/1 -> cfblk52/1
  emi_1479/1 -> cfblk52/2
  cfblk52/1 -> emi_1480/1

== system sampleModel7293_pp_1_1/cfblk53 ==
  emi_43 : Inport
  Action Port : ActionPort  ActionType=then
  cfblk53 : simulink/Discrete/Transfer Fcn First Order  PoleZ=0.95  ICPrevOutput=0.0  DoSatur=off
      settings: SourceProductName=Simulink
  emi_44 : Outport
  wires:
  emi_43/1 -> cfblk53/1
  cfblk53/1 -> emi_44/1

== system sampleModel7293_pp_1_1/cfblk6 ==
  emi_1814 : Inport
  Action Port : ActionPort  ActionType=then
  cfblk6 : simulink/Continuous/PID Controller  Controller=PID  TimeDomain=Discrete-time  SampleTime=1  IntegratorMethod=Forward Euler  FilterMethod=Forward Euler  Form=Parallel  UseFilter=on  ControllerParametersSource=internal  P=1  I=1  D=0  N=100  InitialConditionSource=internal  InitialConditionForIntegrator=0  InitialConditionForFilter=0  ExternalReset=none  LimitOutput=off  UpperSaturationLimit=inf  LowerSaturationLimit=-inf  LinearizeAsGain=off  AntiWindupMode=none  Kb=1  TrackingMode=off  Kt=1  PParamMin=[]  PParamMax=[]  IParamMin=[]  IParamMax=[]  DParamMin=[]  DParamMax=[]  NParamMin=[]  NParamMax=[]  KbParamMin=[]  KbParamMax=[]  KtParamMin=[]  KtParamMax=[]  POutMin=[]  POutMax=[]  IOutMin=[]  IOutMax=[]  DOutMin=[]  DOutMax=[]  NOutMin=[]  NOutMax=[]  KbOutMin=[]  KbOutMax=[]  KtOutMin=[]  KtOutMax=[]  IntegratorOutMin=[]  IntegratorOutMax=[]  FilterOutMin=[]  FilterOutMax=[]  SumOutMin=[]  SumOutMax=[]  SumI1OutMin=[]  SumI1OutMax=[]  SumI2OutMin=[]  SumI2OutMax=[]  SumI3OutMin=[]  SumI3OutMax=[]  SumDOutMin=[]  SumDOutMax=[]  SaturationOutMin=[]  SaturationOutMax=[]  IntegratorContinuousStateAttributes=''  IntegratorStateMustResolveToSignalObject=off  IntegratorRTWStateStorageClass=Auto  FilterContinuousStateAttributes=''  FilterStateMustResolveToSignalObject=off  FilterRTWStateStorageClass=Auto  DifferentiatorICPrevScaledInput=0  DifferentiatorOutMin=[]  DifferentiatorOutMax=[]  FilterDiffOutCoefMin=[]  FilterDiffOutCoefMax=[]  SumDenOutMin=[]  SumDenOutMax=[]  SumNumOutMin=[]  SumNumOutMax=[]  ReciprocalOutMin=[]  ReciprocalOutMax=[]  DivideOutMin=[]  DivideOutMax=[]  TunerSelectOption=Transfer Function Based (PID Tuner App)
  emi_1815 : Outport
  wires:
  emi_1814/1 -> cfblk6/1
  cfblk6/1 -> emi_1815/1

== system sampleModel7293_pp_1_1/cfblk62 ==
  emi_710 : Inport
  emi_711 : Inport  Port=2
  Action Port : ActionPort  ActionType=then
  cfblk62 : Delay  ShowEnablePort=on  SampleTime=1
      settings: InputPortMap=u0,e6
  emi_712 : Outport
  wires:
  emi_710/1 -> cfblk62/1
  emi_711/1 -> cfblk62/2
  cfblk62/1 -> emi_712/1

== system sampleModel7293_pp_1_1/cfblk64 ==
  emi_1107 : Inport
  Action Port : ActionPort  ActionType=then
  cfblk64 : UnitDelay
  emi_1108 : Outport
  wires:
  emi_1107/1 -> cfblk64/1
  cfblk64/1 -> emi_1108/1

== system sampleModel7293_pp_1_1/cfblk66 ==
  emi_1008 : Inport
  Action Port : ActionPort  ActionType=then
  cfblk66 : simulink/Discrete/Transfer Fcn Real Zero  ZeroZ=0.75  ICPrevInput=0.0  DoSatur=off
      settings: SourceProductName=Simulink  SourceProductBaseCode=SL
  emi_1009 : Outport
  wires:
  emi_1008/1 -> cfblk66/1
  cfblk66/1 -> emi_1009/1

== system sampleModel7293_pp_1_1/cfblk68 ==
  emi_2012 : Inport
  Action Port : ActionPort  ActionType=then
  cfblk68 : DiscreteIntegrator  OutDataTypeStr=double  ICPrevOutput=DiscIntNeverNeededParam  ICPrevScaledInput=DiscIntNeverNeededParam
  emi_2013 : Outport
  wires:
  emi_2012/1 -> cfblk68/1
  cfblk68/1 -> emi_2013/1

== system sampleModel7293_pp_1_1/cfblk8 ==
  emi_660 : Inport
  Action Port : ActionPort  ActionType=then
  cfblk8 : simulink/Continuous/PID Controller  Controller=PID  TimeDomain=Discrete-time  SampleTime=1  IntegratorMethod=Forward Euler  FilterMethod=Forward Euler  Form=Parallel  UseFilter=on  ControllerParametersSource=internal  P=1  I=1  D=0  N=100  InitialConditionSource=internal  InitialConditionForIntegrator=0  InitialConditionForFilter=0  ExternalReset=none  LimitOutput=off  UpperSaturationLimit=inf  LowerSaturationLimit=-inf  LinearizeAsGain=off  AntiWindupMode=none  Kb=1  TrackingMode=off  Kt=1  PParamMin=[]  PParamMax=[]  IParamMin=[]  IParamMax=[]  DParamMin=[]  DParamMax=[]  NParamMin=[]  NParamMax=[]  KbParamMin=[]  KbParamMax=[]  KtParamMin=[]  KtParamMax=[]  POutMin=[]  POutMax=[]  IOutMin=[]  IOutMax=[]  DOutMin=[]  DOutMax=[]  NOutMin=[]  NOutMax=[]  KbOutMin=[]  KbOutMax=[]  KtOutMin=[]  KtOutMax=[]  IntegratorOutMin=[]  IntegratorOutMax=[]  FilterOutMin=[]  FilterOutMax=[]  SumOutMin=[]  SumOutMax=[]  SumI1OutMin=[]  SumI1OutMax=[]  SumI2OutMin=[]  SumI2OutMax=[]  SumI3OutMin=[]  SumI3OutMax=[]  SumDOutMin=[]  SumDOutMax=[]  SaturationOutMin=[]  SaturationOutMax=[]  IntegratorContinuousStateAttributes=''  IntegratorStateMustResolveToSignalObject=off  IntegratorRTWStateStorageClass=Auto  FilterContinuousStateAttributes=''  FilterStateMustResolveToSignalObject=off  FilterRTWStateStorageClass=Auto  DifferentiatorICPrevScaledInput=0  DifferentiatorOutMin=[]  DifferentiatorOutMax=[]  FilterDiffOutCoefMin=[]  FilterDiffOutCoefMax=[]  SumDenOutMin=[]  SumDenOutMax=[]  SumNumOutMin=[]  SumNumOutMax=[]  ReciprocalOutMin=[]  ReciprocalOutMax=[]  DivideOutMin=[]  DivideOutMax=[]  TunerSelectOption=Transfer Function Based (PID Tuner App)
  emi_661 : Outport
  wires:
  emi_660/1 -> cfblk8/1
  cfblk8/1 -> emi_661/1

== system sampleModel7293_pp_1_1/cfblk9 ==
  emi_264 : Inport
  emi_265 : Inport  Port=2
  Action Port : ActionPort  ActionType=then
  cfblk9 : Delay  DelayLengthSource=Input port  SampleTime=1
      settings: InputPortMap=u0,p1
  emi_266 : Outport
  wires:
  emi_264/1 -> cfblk9/1
  emi_265/1 -> cfblk9/2
  cfblk9/1 -> emi_266/1

== system sampleModel7293_pp_1_1/emi_1010 ==
  Action Port : ActionPort  ActionType=else
  emi_1011 : Assertion

== system sampleModel7293_pp_1_1/emi_1038 ==
  Action Port : ActionPort  ActionType=else
  emi_1039 : Assertion

== system sampleModel7293_pp_1_1/emi_1109 ==
  Action Port : ActionPort  ActionType=else
  emi_1110 : Assertion

== system sampleModel7293_pp_1_1/emi_1247 ==
  Action Port : ActionPort  ActionType=else
  emi_1248 : Assertion

== system sampleModel7293_pp_1_1/emi_1296 ==
  Action Port : ActionPort  ActionType=else
  emi_1297 : Assertion

== system sampleModel7293_pp_1_1/emi_1339 ==
  Action Port : ActionPort  ActionType=else
  emi_1340 : Assertion

== system sampleModel7293_pp_1_1/emi_1395 ==
  Action Port : ActionPort  ActionType=else
  emi_1396 : Assertion

== system sampleModel7293_pp_1_1/emi_1445 ==
  Action Port : ActionPort  ActionType=else
  emi_1446 : Assertion

== system sampleModel7293_pp_1_1/emi_145 ==
  Action Port : ActionPort  ActionType=else
  emi_146 : Assertion

== system sampleModel7293_pp_1_1/emi_1481 ==
  Action Port : ActionPort  ActionType=else
  emi_1482 : Assertion

== system sampleModel7293_pp_1_1/emi_1517 ==
  Action Port : ActionPort  ActionType=else
  emi_1518 : Assertion

== system sampleModel7293_pp_1_1/emi_1545 ==
  Action Port : ActionPort  ActionType=else
  emi_1546 : Assertion

== system sampleModel7293_pp_1_1/emi_1744 ==
  Action Port : ActionPort  ActionType=else
  emi_1745 : Assertion

== system sampleModel7293_pp_1_1/emi_1788 ==
  Action Port : ActionPort  ActionType=else
  emi_1789 : Assertion

== system sampleModel7293_pp_1_1/emi_1816 ==
  Action Port : ActionPort  ActionType=else
  emi_1817 : Assertion

== system sampleModel7293_pp_1_1/emi_1880 ==
  Action Port : ActionPort  ActionType=else
  emi_1881 : Assertion

== system sampleModel7293_pp_1_1/emi_1915 ==
  Action Port : ActionPort  ActionType=else
  emi_1916 : Assertion

== system sampleModel7293_pp_1_1/emi_2014 ==
  Action Port : ActionPort  ActionType=else
  emi_2015 : Assertion

== system sampleModel7293_pp_1_1/emi_267 ==
  Action Port : ActionPort  ActionType=else
  emi_268 : Assertion

== system sampleModel7293_pp_1_1/emi_331 ==
  Action Port : ActionPort  ActionType=else
  emi_332 : Assertion

== system sampleModel7293_pp_1_1/emi_375 ==
  Action Port : ActionPort  ActionType=else
  emi_376 : Assertion

== system sampleModel7293_pp_1_1/emi_403 ==
  Action Port : ActionPort  ActionType=else
  emi_404 : Assertion

== system sampleModel7293_pp_1_1/emi_438 ==
  Action Port : ActionPort  ActionType=else
  emi_439 : Assertion

== system sampleModel7293_pp_1_1/emi_45 ==
  Action Port : ActionPort  ActionType=else
  emi_46 : Assertion

== system sampleModel7293_pp_1_1/emi_460 ==
  Action Port : ActionPort  ActionType=else
  emi_461 : Assertion

== system sampleModel7293_pp_1_1/emi_467 ==
  Action Port : ActionPort  ActionType=else
  emi_468 : Assertion

== system sampleModel7293_pp_1_1/emi_482 ==
  Action Port : ActionPort  ActionType=else
  emi_483 : Assertion

== system sampleModel7293_pp_1_1/emi_662 ==
  Action Port : ActionPort  ActionType=else
  emi_663 : Assertion

== system sampleModel7293_pp_1_1/emi_705 ==
  Action Port : ActionPort  ActionType=else
  emi_706 : Assertion

== system sampleModel7293_pp_1_1/emi_713 ==
  Action Port : ActionPort  ActionType=else
  emi_714 : Assertion

== system sampleModel7293_pp_1_1/emi_741 ==
  Action Port : ActionPort  ActionType=else
  emi_742 : Assertion

== system sampleModel7293_pp_1_1/emi_755 ==
  Action Port : ActionPort  ActionType=else
  emi_756 : Assertion

== system sampleModel7293_pp_1_1/emi_805 ==
  Action Port : ActionPort  ActionType=else
  emi_806 : Assertion

== system sampleModel7293_pp_1_1/emi_870 ==
  Action Port : ActionPort  ActionType=else
  emi_871 : Assertion

== system sampleModel7293_pp_1_1/emi_884 ==
  Action Port : ActionPort  ActionType=else
  emi_885 : Assertion

== system sampleModel7293_pp_1_1/emi_933 ==
  Action Port : ActionPort  ActionType=else
  emi_934 : Assertion

== system sampleModel7293_pp_1_1/emi_947 ==
  Action Port : ActionPort  ActionType=else
  emi_948 : Assertion

== system sampleModel7293_pp_1_1/cfblk164/cfblk4 ==
  emi_760 : Inport
  Action Port : ActionPort  ActionType=then
  cfblk4 : DiscreteZeroPole  Poles=[0 0.5]  Gain=1  SampleTime=-1
  emi_761 : Outport
  wires:
  emi_760/1 -> cfblk4/1
  cfblk4/1 -> emi_761/1

== system sampleModel7293_pp_1_1/cfblk164/cfblk7 ==
  emi_1614 : Inport
  emi_1615 : Inport  Port=2
  Action Port : ActionPort  ActionType=then
  cfblk7 : Delay  ShowEnablePort=on
      settings: InputPortMap=u0,e6
  emi_1616 : Outport
  wires:
  emi_1614/1 -> cfblk7/1
  emi_1615/1 -> cfblk7/2
  cfblk7/1 -> emi_1616/1

== system sampleModel7293_pp_1_1/cfblk164/emi_1617 ==
  Action Port : ActionPort  ActionType=else
  emi_1618 : Assertion

== system sampleModel7293_pp_1_1/cfblk164/emi_762 ==
  Action Port : ActionPort  ActionType=else
  emi_763 : Assertion

== system sampleModel7293_pp_1_1/cfblk165/cfblk15 ==
  cfblk1 : Inport
  Action Port : ActionPort  ActionType=then
  cfblk10 : DiscreteStateSpace  SampleTime=-1
  cfblk11 : Subsystem  TreatAsAtomicUnit=on
  cfblk12 : Subsystem  TreatAsAtomicUnit=on
  cfblk13 : Subsystem  TreatAsAtomicUnit=on
  cfblk14 : simulink/Discrete/Difference  ICPrevInput=0.0  OutMin=[]  OutMax=[]  OutDataTypeStr=double  OutputDataTypeScalingMode=double  OutDataType=fixdt(1, 16)  OutScaling=2^-10  DoSatur=off
  cfblk3 : DiscreteStateSpace  SampleTime=-1
  cfblk4 : Delay  ShowEnablePort=on
      settings: InputPortMap=u0,e6
  cfblk5 : simulink/Discrete/Transfer Fcn Real Zero  ZeroZ=0.75  ICPrevInput=0.0  DoSatur=off
      settings: SourceProductName=Simulink  SourceProductBaseCode=SL
  cfblk6 : simulink/Continuous/PID Controller  Controller=PID  TimeDomain=Discrete-time  SampleTime=-1  IntegratorMethod=Forward Euler  FilterMethod=Forward Euler  Form=Parallel  UseFilter=on  ControllerParametersSource=internal  P=1  I=1  D=0  N=100  InitialConditionSource=internal  InitialConditionForIntegrator=0  InitialConditionForFilter=0  ExternalReset=none  LimitOutput=off  UpperSaturationLimit=inf  LowerSaturationLimit=-inf  LinearizeAsGain=off  AntiWindupMode=none  Kb=1  TrackingMode=off  Kt=1  PParamMin=[]  PParamMax=[]  IParamMin=[]  IParamMax=[]  DParamMin=[]  DParamMax=[]  NParamMin=[]  NParamMax=[]  KbParamMin=[]  KbParamMax=[]  KtParamMin=[]  KtParamMax=[]  POutMin=[]  POutMax=[]  IOutMin=[]  IOutMax=[]  DOutMin=[]  DOutMax=[]  NOutMin=[]  NOutMax=[]  KbOutMin=[]  KbOutMax=[]  KtOutMin=[]  KtOutMax=[]  IntegratorOutMin=[]  IntegratorOutMax=[]  FilterOutMin=[]  FilterOutMax=[]  SumOutMin=[]  SumOutMax=[]  SumI1OutMin=[]  SumI1OutMax=[]  SumI2OutMin=[]  SumI2OutMax=[]  SumI3OutMin=[]  SumI3OutMax=[]  SumDOutMin=[]  SumDOutMax=[]  SaturationOutMin=[]  SaturationOutMax=[]  IntegratorContinuousStateAttributes=''  IntegratorStateMustResolveToSignalObject=off  IntegratorRTWStateStorageClass=Auto  FilterContinuousStateAttributes=''  FilterStateMustResolveToSignalObject=off  FilterRTWStateStorageClass=Auto  DifferentiatorICPrevScaledInput=0  DifferentiatorOutMin=[]  DifferentiatorOutMax=[]  FilterDiffOutCoefMin=[]  FilterDiffOutCoefMax=[]  SumDenOutMin=[]  SumDenOutMax=[]  SumNumOutMin=[]  SumNumOutMax=[]  ReciprocalOutMin=[]  ReciprocalOutMax=[]  DivideOutMin=[]  DivideOutMax=[]  TunerSelectOption=Transfer Function Based (PID Tuner App)
  cfblk7 : DiscreteTransferFcn
  cfblk8 : Delay  ShowEnablePort=on
      settings: InputPortMap=u0,e6
  cfblk9 : Delay
  cyemi_{57..70} (14 alike) : DataTypeConversion  OutDataTypeStr=double
  emi_1024 : Subsystem  TreatAsAtomicUnit=on
  emi_1026 : If  IfExpression=Inf <= u1
  emi_1027 : DataTypeConversion  OutDataTypeStr=double
  emi_1410 : Subsystem  TreatAsAtomicUnit=on
  emi_1412 : If  IfExpression=Inf <= u1
  emi_1413 : DataTypeConversion  OutDataTypeStr=double
  emi_1766 : Subsystem  TreatAsAtomicUnit=on
  emi_1768 : If  IfExpression=Inf <= u1
  emi_1769 : DataTypeConversion  OutDataTypeStr=double
  cfblk2 : Outport
  cfblk15 : Outport  Port=2
  wires:
  cfblk14/1 -> cyemi_58/1, cyemi_63/1
  cfblk3/1 -> cfblk2/1
  cfblk6/1 -> cyemi_65/1, cyemi_68/1
  cyemi_57/1 -> cfblk10/1
  cfblk7/1 -> cyemi_57/1, emi_1413/1
  cfblk9/1 -> cyemi_60/1
  cyemi_61/1 -> cfblk14/1
  cfblk1/1 -> cyemi_61/1
  cyemi_62/1 -> cfblk3/1
  cfblk10/1 -> cyemi_62/1
  cyemi_63/1 -> cfblk4/1
  cyemi_64/1 -> cfblk4/2
  cfblk5/1 -> cyemi_64/1
  cyemi_65/1 -> cfblk5/1
  cyemi_66/1 -> cfblk6/1
  cyemi_67/1 -> cfblk7/1
  cfblk8/1 -> cyemi_67/1, emi_1027/1, emi_1769/1
  cyemi_68/1 -> cfblk8/1
  cyemi_69/1 -> cfblk8/2
  cyemi_70/1 -> cfblk9/1
  cfblk4/1 -> cyemi_70/1
  cyemi_58/1 -> cfblk11/1(emi_1022)
  cfblk11/1(emi_1023) -> cyemi_69/1, cyemi_59/1
  emi_1026/1 -> cfblk11/Action
  emi_1026/2 -> emi_1024/Action
  emi_1027/1 -> emi_1026/1
  cyemi_59/1 -> cfblk12/1(emi_1408)
  cfblk12/1(emi_1409) -> cyemi_66/1
  emi_1412/1 -> cfblk12/Action
  emi_1412/2 -> emi_1410/Action
  emi_1413/1 -> emi_1412/1
  cyemi_60/1 -> cfblk13/1(emi_1764)
  cfblk13/1(emi_1765) -> cfblk15/1
  emi_1768/1 -> cfblk13/Action
  emi_1768/2 -> emi_1766/Action
  emi_1769/1 -> emi_1768/1

== system sampleModel7293_pp_1_1/cfblk165/cfblk16 ==
  cfblk1 : Inport
  Action Port : ActionPort  ActionType=else
  cfblk10 : simulink/Discrete/Tapped Delay  vinit=0.0  samptime=-1  NumDelays=1  DelayOrder=Oldest  includeCurrent=off
  cfblk11 : Subsystem  TreatAsAtomicUnit=on
  cfblk12 : Subsystem  TreatAsAtomicUnit=on
  cfblk13 : DiscreteTransferFcn
  cfblk14 : DiscreteStateSpace  SampleTime=-1
  cfblk{4,9,16..17} (4 alike) : Delay
  cfblk3 : DiscreteIntegrator  SampleTime=-1  OutDataTypeStr=double  ICPrevOutput=DiscIntNeverNeededParam  ICPrevScaledInput=DiscIntNeverNeededParam
  cfblk5 : UnitDelay  SampleTime=-1
  cfblk6 : DiscreteTransferFcn
  cfblk7 : DiscreteTransferFcn
  cfblk8 : Subsystem  TreatAsAtomicUnit=on
  cyemi_{72..86} (15 alike) : DataTypeConversion  OutDataTypeStr=double
  emi_1160 : Subsystem  TreatAsAtomicUnit=on
  emi_1162 : If  IfExpression=0 <= u1
  emi_1163 : DataTypeConversion  OutDataTypeStr=double
  emi_152 : Subsystem  TreatAsAtomicUnit=on
  emi_154 : If  IfExpression=0 <= u1
  emi_155 : DataTypeConversion  OutDataTypeStr=double
  emi_2077 : Subsystem  TreatAsAtomicUnit=on
  emi_2079 : If  IfExpression=0 <= u1
  emi_2080 : DataTypeConversion  OutDataTypeStr=double
  cfblk2 : Outport
  cfblk15 : Outport  Port=2
  wires:
  cfblk14/1 -> cfblk2/1
  cfblk9/1 -> cyemi_73/1, cyemi_81/1
  cyemi_72/1 -> cfblk10/1
  cfblk6/1 -> cyemi_74/1, cyemi_75/1
  cyemi_76/1 -> cfblk13/1
  cfblk1/1 -> cyemi_76/1
  cyemi_77/1 -> cfblk14/1
  cyemi_78/1 -> cfblk16/1
  cfblk5/1 -> cyemi_78/1, emi_2080/1
  cyemi_79/1 -> cfblk17/1
  cfblk7/1 -> cyemi_79/1
  cyemi_80/1 -> cfblk3/1
  cfblk16/1 -> cyemi_80/1
  cyemi_81/1 -> cfblk4/1
  cyemi_82/1 -> cfblk5/1
  cfblk4/1 -> cyemi_82/1
  cyemi_83/1 -> cfblk6/1
  cfblk17/1 -> cyemi_83/1, emi_1163/1
  cyemi_84/1 -> cfblk7/1
  cfblk10/1 -> cyemi_84/1
  cfblk13/1 -> cyemi_85/1
  cyemi_86/1 -> cfblk9/1
  cfblk3/1 -> cyemi_86/1, emi_155/1
  cyemi_73/1 -> cfblk11/1(emi_150)
  cfblk11/1(emi_151) -> cyemi_77/1
  emi_154/1 -> cfblk11/Action
  emi_154/2 -> emi_152/Action
  emi_155/1 -> emi_154/1
  cyemi_74/1 -> cfblk12/1(emi_1157)
  cyemi_75/1 -> cfblk12/2(emi_1158)
  cfblk12/1(emi_1159) -> cyemi_72/1
  emi_1162/1 -> cfblk12/Action
  emi_1162/2 -> emi_1160/Action
  emi_1163/1 -> emi_1162/1
  cyemi_85/1 -> cfblk8/1(emi_2075)
  cfblk8/1(emi_2076) -> cfblk15/1
  emi_2079/1 -> cfblk8/Action
  emi_2079/2 -> emi_2077/Action
  emi_2080/1 -> emi_2079/1

== system sampleModel7293_pp_1_1/cfblk165/cfblk5 ==
  emi_2098 : Inport
  Action Port : ActionPort  ActionType=then
  cfblk5 : DiscreteZeroPole  Poles=[0 0.5]  Gain=1  SampleTime=-1
  emi_2099 : Outport
  wires:
  emi_2098/1 -> cfblk5/1
  cfblk5/1 -> emi_2099/1

== system sampleModel7293_pp_1_1/cfblk165/cfblk6 ==
  emi_115 : Inport
  Action Port : ActionPort  ActionType=then
  cfblk6 : DiscreteZeroPole  Poles=[0 0.5]  Gain=1  SampleTime=-1
  emi_116 : Outport
  wires:
  emi_115/1 -> cfblk6/1
  cfblk6/1 -> emi_116/1

== system sampleModel7293_pp_1_1/cfblk165/emi_117 ==
  Action Port : ActionPort  ActionType=else
  emi_118 : Assertion

== system sampleModel7293_pp_1_1/cfblk165/emi_2100 ==
  Action Port : ActionPort  ActionType=else
  emi_2101 : Assertion

== system sampleModel7293_pp_1_1/cfblk166/cfblk5 ==
  emi_1693 : Inport
  Action Port : ActionPort  ActionType=then
  cfblk5 : DiscreteFir
  emi_1694 : Outport
  wires:
  emi_1693/1 -> cfblk5/1
  cfblk5/1 -> emi_1694/1

== system sampleModel7293_pp_1_1/cfblk166/cfblk7 ==
  emi_1836 : Inport
  Action Port : ActionPort  ActionType=then
  cfblk7 : simulink/Discrete/Difference  ICPrevInput=0.0  OutMin=[]  OutMax=[]  OutDataTypeStr=double  OutputDataTypeScalingMode=double  OutDataType=fixdt(1, 16)  OutScaling=2^-10  DoSatur=off
  emi_1837 : Outport
  wires:
  emi_1836/1 -> cfblk7/1
  cfblk7/1 -> emi_1837/1

== system sampleModel7293_pp_1_1/cfblk166/emi_1695 ==
  Action Port : ActionPort  ActionType=else
  emi_1696 : Assertion

== system sampleModel7293_pp_1_1/cfblk166/emi_1838 ==
  Action Port : ActionPort  ActionType=else
  emi_1839 : Assertion
